simulink model "HW3_Q2"  (R2022b)
settings: Solver=FixedStepDiscrete  StartTime=0.0  StopTime=20  FixedStep=1  RelTol=1e-3  EnableMultiTasking=on
settings Model: Creator=Erfan  LastModifiedBy=Erfan
settings SolverCC: AlgebraicLoopSolver=TrustRegion  AutoInsertRateTranBlk=on
settings OptimizationCC: LifeSpan=inf
settings DebuggingCC: UnconnectedInputMsg=warning  UnconnectedOutputMsg=warning  UnconnectedLineMsg=warning  SFUnexpectedBacktrackingDiag=warning  SFNoUnconditionalDefaultTransitionDiag=warning  SFExecutionAtInitializationDiag=none  ArithmeticOperatorsInVariantConditions=warning
settings ModelReferenceCC: EnableRefExpFcnMdlSchedulingChecks=on
settings SFSimCC: SimUseLocalCustomCode=off  CustomCodeUndefinedFunction=UseInterfaceOnly
settings RTWCC: RTWUseLocalCustomCode=off  DLArmComputeVersion=19.05
settings CodeAppCC: StateflowObjectComments=on
settings GRTTargetCC: TargetLangStandard=C89/C90 (ANSI)
settings ConfigComp: CovMetricSettings=dw  CovSaveCumulativeToWorkspaceVar=on  CovSaveSingleToWorkspaceVar=on  CovExternalEMLEnable=off

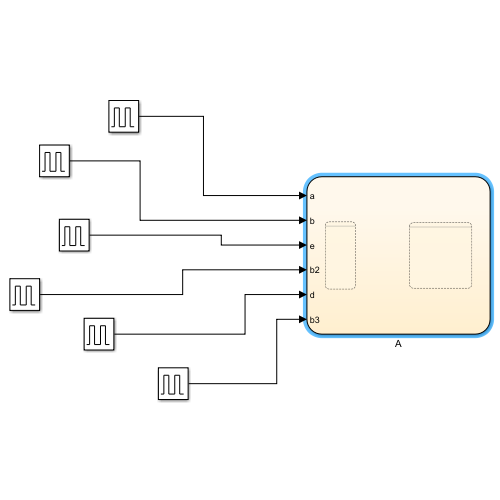
[thumbnail: Simulink's stored preview of the top-level diagram]
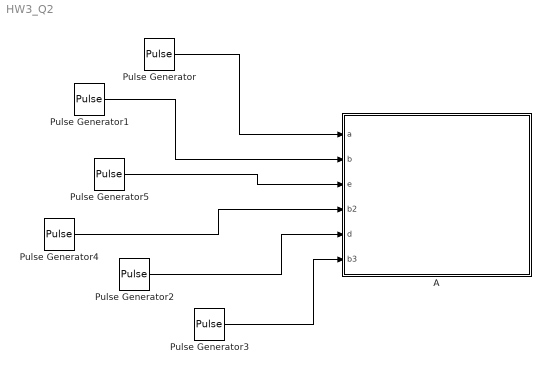
== system HW3_Q2 ==
  A : Stateflow chart  TreatAsAtomicUnit=on
      settings: PortSchema="{\"entries\":[{\"content\":{\"sides\":[{\"content\":{\"connectorIds\":[\"In1\",\"In5\",\"In2\",\"In4\",\"In3\",\"In6\"]},\"type\":\"ConnectorPlacement.EquallySpacedRectSide\",\"uuid\":\"a707456b-31f5-4953-91fb-0fbd89df4214\"},{\"content\":{\"connectorIds\":[],\"side\":\"RIGHT\"},\"type\":\"ConnectorPlacement.EquallySpacedRectSide\",\"uuid\":\"3ac9d269-bd3e-44d3-a73f-27f2f71459d3\"},{\"content\":{\"connectorIds\":[],\"side\":\"TOP\"},\"type\":\"ConnectorPlacement.EquallySpacedRectSide\",\"uuid\":\"e692d9e1-56f5-48c0-9185-308d4fa4ebb2\"}]},\"type\":\"ConnectorPlacement.EquallySpacedConnector\",\"uuid\":\"798245d0-d1b4-435a-bfb4-da874f9fcc94\"}],\"packageUris\":[\"http://schema.mathworks.com/mf0/Connector/R2020b\"],\"version\":\"1.0\"}"
  Pulse Generator : DiscretePulseGenerator  PulseType=Time based  Period=100  PhaseDelay=2
  Pulse Generator1 : DiscretePulseGenerator  PulseType=Time based  Period=100  PhaseDelay=4
  Pulse Generator2 : DiscretePulseGenerator  PulseType=Time based  Period=100  PhaseDelay=10
  Pulse Generator3 : DiscretePulseGenerator  PulseType=Time based  Period=100  PhaseDelay=12
  Pulse Generator4 : DiscretePulseGenerator  PulseType=Time based  Period=100  PhaseDelay=8
  Pulse Generator5 : DiscretePulseGenerator  PulseType=Time based  Period=100  PhaseDelay=6
  wires:
  Pulse Generator/1 -> A/1(a)
  Pulse Generator1/1 -> A/5(b)
  Pulse Generator5/1 -> A/2(e)
  Pulse Generator4/1 -> A/4(b2)
  Pulse Generator2/1 -> A/3(d)
  Pulse Generator3/1 -> A/6(b3)

== stateflow chart HW3_Q2/A ==
  state B [parallel]
    settings: executionOrder=1
    state State_1
    state State_2
    (default) -> State_1
    State_1 -> State_2 : [c]
    State_2 -> State_1 : [(b || b2 || b3) && in(C.D.D2)]
  state C [parallel]
    settings: executionOrder=2
    state D
      state D1
      state D2
      (default) -> D1
      D1 -> D2 : [e]{c = 0;}
      D2 -> D2 : [e]
    state G
    G -> D : [a]{c = 1;}
    (default) -> G
    D -> G : [d]
  data: a input; e input; d input; b2 input; b input; c local =0; b3 input
